simulink library "visionsources"  (R2017b)
settings: Solver=ode45  StartTime=0.0  StopTime=10.0  RelTol=1e-3
undefined symbols (not defined in the file or in its folder): checker_board
libraries: dspvision x1
settings Model: ExtModeAutoUpdateStatusClock=off  Creator=The MathWorks, Inc.  LastModifiedBy=The MathWorks, Inc.
settings DataIOCC: LimitDataPoints=on  SaveFormat=Array  SignalLoggingSaveFormat=ModelDataLogs
settings OptimizationCC: BlockReduction=off  BooleanDataType=off  ExpressionDepthLimit=2147483647  LifeSpan=inf
settings DebuggingCC: SaveWithParameterizedLinksMsg=none  UnderspecifiedInitializationDetection=Classic  MergeDetectMultiDrivingBlocksExec=none  SignalResolutionControl=TryResolveAllWithWarning  FcnCallInpInsideContextMsg=warning  StateNameClashWarn=warning  StrictBusMsg=Warning  SFUnexpectedBacktrackingDiag=warning  SFNoUnconditionalDefaultTransitionDiag=warning  SFExecutionAtInitializationDiag=none
settings HardwareCC: ProdBitPerPointer=32  ProdBitPerSizeT=32  ProdBitPerPtrDiffT=32  ProdLargestAtomicFloat=None  ProdIntDivRoundTo=Undefined  ProdEndianess=Unspecified  ProdWordSize=32  ProdHWDeviceType=32-bit Generic  TargetUnknown=on
settings ModelReferenceCC: PropagateSignalLabelsOutOfModel=off
settings CodeAppCC: StateflowObjectComments=on
settings GRTTargetCC: TargetLangStandard=C89/C90 (ANSI)  GeneratePreprocessorConditionals=Disable all  CombineOutputUpdateFcns=off  GRTInterface=on
settings ConfigComp: CovMetricSettings=dw  CovHtmlReporting=on  CovSaveCumulativeToWorkspaceVar=on  CovSaveSingleToWorkspaceVar=on  CovExternalEMLEnable=off

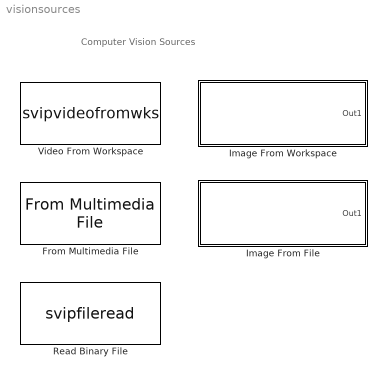
== system visionsources ==
  note: Computer Vision Sources
  From Multimedia File : dspvision/From Multimedia File  inputFilename=vipmen.avi  loop=on  numPlays=inf  outputStreams=Video only  videoDataType=single  audioDataType=int16  inheritSampleTime=on  userDefinedSampleTime=1/30  noAudioOutput=off  isIntensityVideo=off  fourcc=RGB  colorVideoFormat=One multidimensional signal  outputEOF=off  dataOrg=Column-major  audioFrameSize=1024  computeAudioFrameSize=off  outSamplingMode=Sample based
      settings: SourceProductBaseCode=VP
  Image From File : Subsystem  Tag=vipblks_nd  DialogController=vipDDGCreate  mask(Image From File){FileName=peppers.png, imagePorts=One multidimensional signal, Ts=inf, ImageDataType=Inherit from input image, Signed=on, WordLength=16, sdImageDataType=uint(8), FractionLengthMode=User-defined, FractionLength=15, OutPortLabels=R|G|B}
      mask prompts: FileName "vision:masks:FileName_MP"; imagePorts "vision:masks:ImageSignal"; Ts "vision:masks:SampleTime"; ImageDataType "vision:masks:OutputDataType"; Signed "dspshared:FixptDialog:signed"; WordLength "vision:masks:WordLength"; sdImageDataType "vision:masks:UserdefinedDataType"; FractionLengthMode "vision:masks:SetFractionLengthInOutputTo"; FractionLength "vision:masks:FractionLength"; OutPortLabels "vision:masks:OutputPortLabels"
      mask help: vision:masks:ImageFromFileDescription
      mask init:
      | vipblks_nd_compatible;
      | [v, namechange]=vipblkimsrc(1, '',0,FileName);
      | ImageValue = v;
      | vipblkimsrc(2, v, namechange,FileName);
      mask Help: eval('visionblockhelp;')
      mask TypeOptions imagePorts: vision:masks:OneMultidimensionalSignal | vision:masks:SeparateColorSignals
      mask Callback imagePorts: vipblkimsrc(-1);
      mask TypeOptions ImageDataType: double | single | int8 | uint8 | int16 | uint16 | int32 | uint32 | boolean | vision:masks:Fixedpoint | vision:masks:Userdefined | vision:masks:InheritFromInputImage | vision:masks:InheritViaBackPropagation
      mask TypeOptions FractionLengthMode: vision:masks:BestPrecision | vision:masks:Userdefined
      mask DialogControl ParameterTabVar0 Prompt: Main
      mask DialogControl FileName Prompt: File Name:
      mask DialogControl imagePorts Prompt: Image signal:
      mask DialogControl Ts Prompt: Sample time:
      mask DialogControl ImageDataType Prompt: Output data type:
      mask DialogControl WordLength Prompt: Word length:
      mask DialogControl sdImageDataType Prompt: User-defined data type (e.g. sfix(16), uint(8), float('single')):
      mask DialogControl FractionLengthMode Prompt: Set fraction length in output to:
      mask DialogControl FractionLength Prompt: Fraction length:
      mask DialogControl OutPortLabels Prompt: Output port labels:
      mask Display: disp('peppers.png');port_label('output',1,'Image');
  Image From Workspace : Subsystem  Tag=vipblks_nd  mask(Image From Workspace){ImageValue=checker_board(10), Ts=inf, imagePorts=One multidimensional signal, OutPortLabels=R|G|B, ImageDataType=Inherit from 'Value', Signed=on, WordLength=16, sdImageDataType=sfix(16), FractionLengthMode=User-defined, FractionLength=15}
      mask prompts: ImageValue "vision:masks:Value"; Ts "vision:masks:SampleTime"; imagePorts "vision:masks:ImageSignal"; OutPortLabels "vision:masks:OutputPortLabels"; ImageDataType "vision:masks:OutputDataType"; Signed "vision:masks:Signed"; WordLength "vision:masks:WordLength"; sdImageDataType "vision:masks:UserdefinedDataType"; FractionLengthMode "vision:masks:SetFractionLengthInOutputTo"; FractionLength "vision:masks:FractionLength"
      mask help: vision:masks:ImageFromWorkspaceDescription
      mask init:
      | ImageVal = get_param(gcbh, 'ImageValue');
      | vipblks_nd_compatible;
      | [v,namechange]=vipblkimsrc(1, ImageValue, 0,'');
      | vipblkimsrc(2, v, namechange,'');
      mask Help: eval('visionblockhelp;')
      mask TypeOptions imagePorts: vision:masks:OneMultidimensionalSignal | vision:masks:SeparateColorSignals
      mask Callback imagePorts: vipblkimsrc(-1);
      mask TypeOptions ImageDataType: double | single | int8 | uint8 | int16 | uint16 | int32 | uint32 | boolean | vision:masks:Fixedpoint | vision:masks:Userdefined | vision:masks:InheritFromValue | vision:masks:InheritViaBackPropagation
      mask Callback ImageDataType: vipblkimsrc(-1, 1);
      mask Callback sdImageDataType: vipblkimsrc(-1);
      mask TypeOptions FractionLengthMode: vision:masks:BestPrecision | vision:masks:Userdefined
      mask Callback FractionLengthMode: vipblkimsrc(-1, 1);
      mask DialogControl ParameterTabVar0 Prompt: dspshared:FixptDialog:main
      mask DialogControl ImageValue Prompt: Value:
      mask DialogControl Ts Prompt: Sample time:
      mask DialogControl imagePorts Prompt: Image signal:
      mask DialogControl OutPortLabels Prompt: Output port labels:
      mask DialogControl ParameterTabVar01 Prompt: dspshared:FixptDialog:dataTypes
      mask DialogControl ImageDataType Prompt: Output data type:
      mask DialogControl WordLength Prompt: Word length:
      mask DialogControl sdImageDataType Prompt: User-defined data type (e.g. sfix(16), uint(8), float('single')):
      mask DialogControl FractionLengthMode Prompt: Set fraction length in output to:
      mask DialogControl FractionLength Prompt: Fraction length:
      mask Display: disp(ImageVal);port_label('output',1,'Image');
  Read Binary File : S-Function  DialogController=vipDDGCreate  FunctionName=svipfileread  Parameters=FileName, loopOrNot, numLoops, VideoFormat, FOURCC, BitStreamFormat, NumOutputs, Bits, ComponentOrder, Interlaced, LineOrdering, FrameSizes, PackFrameSize, SignedOutput, FileEndian, OutputEOF,Ts  SFunctionDeploymentMode=off  EnableBusSupport=off  mask(Read Binary File){FileName=vipmen.bin, loopOrNot=on, numLoops=1, VideoFormat=Four character codes, FOURCC=I420, BitStreamFormat=Planar, NumOutputs=3, ComponentOrder=[1 2 3], Interlaced=off, LineOrdering=Top line first, Ts=1/30, Component1=Y', Component2=Cb, Component3=Cr, Component4=Alpha, Bits1=8, Bits2=8, Bits3=8, Bits4=8, Rows1=120, Rows2=60, Rows3=60, Rows4=288, Cols1=160, Cols2=80, Cols3=80, Cols4=352, YRows=120, YCols=160, SignedOutput=off, FileEndian=Little endian, OutputEOF=off}
      mask prompts: FileName "vision:masks:FileName"; loopOrNot "vision:masks:Loop"; numLoops "vision:masks:NumberOfTimesToPlayFile"; VideoFormat "vision:masks:VideoFormat"; FOURCC "vision:masks:VideoFileFormatLabel"; BitStreamFormat "vision:masks:BitStreamFormat"; NumOutputs "vision:masks:NumberOfOutputs"; ComponentOrder "vision:masks:ComponentOrderInBitStreamEgYCbCr"; Interlaced "vision:masks:InterlacedVideo"; LineOrdering "vision:masks:LineOrdering"; Ts "vision:masks:SampleTime"; Component1 "vision:masks:Component1_1"; Component2 "vision:masks:Component2_1"; Component3 "vision:masks:Component3_1"; Component4 "vision:masks:Component4_1"; Bits1 "vision:masks:Bits1"; Bits2 "vision:masks:Bits2"; Bits3 "vision:masks:Bits3"; Bits4 "vision:masks:Bits4"; Rows1 "vision:masks:Rows1"; Rows2 "vision:masks:Rows2"; Rows3 "vision:masks:Rows3"; Rows4 "vision:masks:Rows4"; Cols1 "vision:masks:Cols1"; Cols2 "vision:masks:Cols2"; Cols3 "vision:masks:Cols3"; Cols4 "vision:masks:Cols4"; YRows "vision:masks:SizeOfYCompoenetRows"; YCols "vision:masks:SizeOfYComponentCols"; SignedOutput "vision:masks:InputFileHasSignedData_1"; FileEndian "vision:masks:ByteOrderInBinaryFile"; OutputEOF "vision:masks:OutputEndoffileIndicator_1"
      mask help: vision:masks:ReadBinaryFileDescription
      mask init:
      | Rows = {Rows1 Rows2 Rows3 Rows4};
      | Cols = {Cols1 Cols2 Cols3 Cols4};
      | Bits = {Bits1 Bits2 Bits3 Bits4};
      | Components = {Component1 Component2 Component3 Component4};
      | videoformat = get_param(gcb, 'VideoFormat');
      | bitstreamformat = get_param(gcb, 'BitStreamFormat');
      | fourcc = get_param(gcb, 'FOURCC');
      | outputeof = get_param(gcb, 'OutputEOF');
      | [FrameSizes, PackFrameSize, FOURCC, NumOutputs,...
      |     maskdisplay, Bits, FileName] =...
      |     vipblkreadbinaryfile(NumOutputs, Components, ComponentOrder,...
      |     Rows, Cols, YRows, YCols, Bits, FileName, videoformat, ...
      |     bitstreamformat, fourcc, outputeof);
      | ComponentOrder = ComponentOrder - 1;
      | set_param(gcb, 'MaskDisplay', maskdisplay);
      mask Help: eval('visionblockhelp;')
      mask TypeOptions VideoFormat: vision:masks:FourCharacterCodes | vision:masks:Custom
      mask TypeOptions FOURCC: AYUV | CLJR | cyuv | GREY | I420 | IF09 | IMC1 | IMC2 | IMC3 | IMC4 | IUYV | IY41 | IYU1 | IYU2 | IYUV | NV12 | NV21 | UYNV | UYVY | V210 | Y411 | Y41P | Y41T | Y422 | Y42T | Y8 | Y800 | YUNV | YUY2 | YUYV | YV12 | YV16 | YVU9 | YVYU
      mask TypeOptions BitStreamFormat: vision:masks:Packed | vision:masks:Planar
      mask TypeOptions NumOutputs: 1 | 2 | 3 | 4
      mask TypeOptions LineOrdering: vision:masks:TopLineFirst | vision:masks:BottomLineFirst
      mask TypeOptions FileEndian: vision:masks:LittleEndian | vision:masks:BigEndian
      mask Display: disp('vipmen.bin');port_label('output', 1,'Y''');port_label('output', 2,'Cb');port_label('output', 3,'Cr');
  Video From Workspace : S-Function  FunctionName=svipvideofromwks  Parameters=signal,Ts, finaloutActive,imagePorts, finalout  SFunctionDeploymentMode=off  EnableBusSupport=off  mask(Video From Workspace){signal=rand(32,32,3,5), Ts=1, finalout=Obsolete, finaloutActive=Setting to zero, imagePorts=One multidimensional signal, OutPortLabels=R|G|B}
      mask prompts: signal "vision:masks:Signal"; Ts "vision:masks:SampleTime"; finalout "vision:masks:FormOutputAfterFinalValue"; finaloutActive "vision:masks:FormOutputAfterFinalValueBy"; imagePorts "vision:masks:ImageSignal"; OutPortLabels "vision:masks:OutputPortLabels"
      mask help: vision:masks:VideoFromWorkspaceDescription
      mask init:
      | signalValue = get_param(gcbh, 'signal');
      | vipblkvideofromws(signal);
      mask Help: eval('visionblockhelp;')
      mask TypeOptions finalout: vision:masks:SettingToZero | vision:masks:HoldingFinalValue | vision:masks:CyclicRepetition | vision:masks:Obsolete
      mask TypeOptions finaloutActive: vision:masks:SettingToZero | vision:masks:HoldingFinalValue | vision:masks:CyclicRepetition
      mask TypeOptions imagePorts: vision:masks:OneMultidimensionalSignal | vision:masks:SeparateColorSignals
      mask Callback imagePorts: vipblkvideofromws
      mask Display:
      | disp(get_param(gcbh, 'signal'));
      | port_label('output',1,'Image');

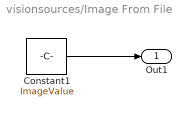
== system visionsources/Image From File ==
  Constant1 : Constant  Value=ImageValue  SampleTime=Ts
  Out1 : Outport
  wires:
  Constant1/1 -> Out1/1

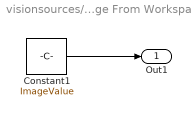
== system visionsources/Image From Workspace ==
  Constant1 : Constant  Value=ImageValue  SampleTime=Ts
  Out1 : Outport
  wires:
  Constant1/1 -> Out1/1
